simulink model "ackerman_ROS_neural_controller_v2"  (R2023a)
settings: Solver=FixedStepDiscrete  StartTime=0.0  StopTime=200  FixedStep=0.1  RelTol=1e-3
undefined symbols (not defined in the file or in its folder): Angular, Linear
libraries: neural x413, robotlib x15, robotcorelib x1
(part 15 of 17)

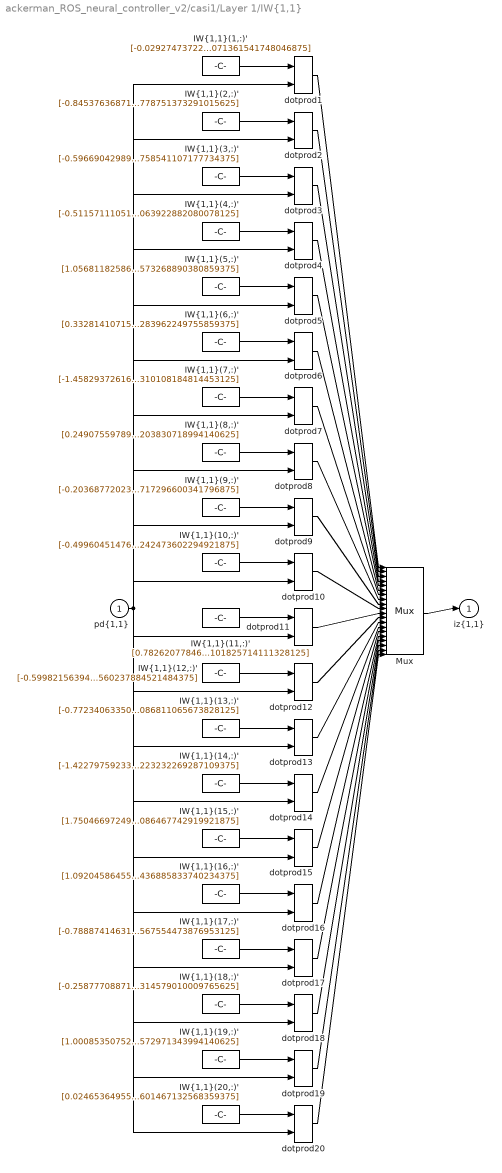
== system ackerman_ROS_neural_controller_v2/casi1/Layer 1/IW{1,1} ==
  "pd{1,1}" : Inport  PortDimensions=8  SampleTime=0.1
      mask Display: e = 0.06;c1 = [120 230 180]/255;c2 = ([120 230 180]+0)/(256+128);c3 = ([120 230 180]+128)/(256+128);patch([0 1 1 0],[0 0 1 1],c1);patch([0 1 1 1-e 1-e 0+e],[0 0 1 1-e 0+e 0+e],c2);patch([0 0 1 1-e 0+e 0+e],[0 1 1 1-e 1-e 0+e],c3);plot([0 1 1 0 0],[0 0 1 1 0]);
  "IW{1,1}(1,:)'" : Constant  Value=[-0.029274737222208684073176954143491457216441631317138671875;-1.0490069849334577867239204351790249347686767578125;-1.018709890416383156974688972695730626583099365234375;0.51758057561495485199287713840021751821041107177734375;-0.49421140001316643530770988945732824504375457763671875;-1.148479697189265014145576060400344431400299072265625;-0.1589169134791238169324145701466477476060390472412109375;-0.12069391049774129409666301171455415897071361541748046875]
      mask Display: e = 0.06;c1 = [120 150 230]/255;c2 = ([120 150 230]+0)/383;c3 = ([120 150 230]+128)/383;patch([0 1 1 0],[0 0 1 1],c1);patch([0 1 1 1-e 1-e 0+e],[0 0 1 1-e 0+e 0+e],c2);patch([0 0 1 1-e 0+e 0+e],[0 1 1 1-e 1-e 0+e],c3);plot([0 1 1 0 0],[0 0 1 1 0]);disp('Weights');
  "IW{1,1}(10,:)'" : Constant  Value=[-0.49960451476214462473990352009423077106475830078125;0.84481568535207518522156533435918390750885009765625;0.328484535401980470847860260619199834764003753662109375;1.38195060372174882701301612542010843753814697265625;-1.020587480316577977390579690109007060527801513671875;-1.05782819768129865423134106094948947429656982421875;-1.038884014221790774712417260161601006984710693359375;-0.5820201999400473891199681020225398242473602294921875]
      mask Display: e = 0.06;c1 = [120 150 230]/255;c2 = ([120 150 230]+0)/383;c3 = ([120 150 230]+128)/383;patch([0 1 1 0],[0 0 1 1],c1);patch([0 1 1 1-e 1-e 0+e],[0 0 1 1-e 0+e 0+e],c2);patch([0 0 1 1-e 0+e 0+e],[0 1 1 1-e 1-e 0+e],c3);plot([0 1 1 0 0],[0 0 1 1 0]);disp('Weights');
  "IW{1,1}(11,:)'" : Constant  Value=[0.78262077846378497181234479285194538533687591552734375;1.506770310513398936080875500920228660106658935546875;0.86605393694049992436845286647439934313297271728515625;0.0785178721101223719980310988830751739442348480224609375;-0.2140063053068555765090508202774799428880214691162109375;-2.454262585311906885721100479713641107082366943359375;1.6946832898832386860021870234049856662750244140625;-0.38077853428415864289746650683810003101825714111328125]
      mask Display: e = 0.06;c1 = [120 150 230]/255;c2 = ([120 150 230]+0)/383;c3 = ([120 150 230]+128)/383;patch([0 1 1 0],[0 0 1 1],c1);patch([0 1 1 1-e 1-e 0+e],[0 0 1 1-e 0+e 0+e],c2);patch([0 0 1 1-e 0+e 0+e],[0 1 1 1-e 1-e 0+e],c3);plot([0 1 1 0 0],[0 0 1 1 0]);disp('Weights');
  "IW{1,1}(12,:)'" : Constant  Value=[-0.599821563945515112692419279483146965503692626953125;-1.2038921753291866867385806472157128155231475830078125;0.1467090791546092898300912565900944173336029052734375;-0.9339192656969517170040262499242089688777923583984375;-1.9352619442102187985454975205357186496257781982421875;0.423900644271696436238272553964634425938129425048828125;-0.2311222652018269096974023568691336549818515777587890625;-0.432161927375341592405533219789504073560237884521484375]
      mask Display: e = 0.06;c1 = [120 150 230]/255;c2 = ([120 150 230]+0)/383;c3 = ([120 150 230]+128)/383;patch([0 1 1 0],[0 0 1 1],c1);patch([0 1 1 1-e 1-e 0+e],[0 0 1 1-e 0+e 0+e],c2);patch([0 0 1 1-e 0+e 0+e],[0 1 1 1-e 1-e 0+e],c3);plot([0 1 1 0 0],[0 0 1 1 0]);disp('Weights');
  "IW{1,1}(13,:)'" : Constant  Value=[-0.77234063350789605717494623604579828679561614990234375;-0.678866375462015891883993390365503728389739990234375;0.520805280323371366790752290398813784122467041015625;0.59851454718035934643438622515532188117504119873046875;-0.138405727580928117337322191815474070608615875244140625;-1.41761697214059267935226671397686004638671875;0.7043140607950550968752168046194128692150115966796875;-0.2470794229904558492183497264704783447086811065673828125]
      mask Display: e = 0.06;c1 = [120 150 230]/255;c2 = ([120 150 230]+0)/383;c3 = ([120 150 230]+128)/383;patch([0 1 1 0],[0 0 1 1],c1);patch([0 1 1 1-e 1-e 0+e],[0 0 1 1-e 0+e 0+e],c2);patch([0 0 1 1-e 0+e 0+e],[0 1 1 1-e 1-e 0+e],c3);plot([0 1 1 0 0],[0 0 1 1 0]);disp('Weights');
  "IW{1,1}(14,:)'" : Constant  Value=[-1.4227975923300253402459247809019871056079864501953125;0.2249135113468267721525961633233237080276012420654296875;-0.11069963821488136568316207331008627079427242279052734375;-0.287756824738865824020450645548407919704914093017578125;-0.2221314694261346256443090396714978851377964019775390625;0.87249899572179823170614554328494705259799957275390625;1.55828917261681088035629727528430521488189697265625;-0.27320712988680317945267006507492624223232269287109375]
      mask Display: e = 0.06;c1 = [120 150 230]/255;c2 = ([120 150 230]+0)/383;c3 = ([120 150 230]+128)/383;patch([0 1 1 0],[0 0 1 1],c1);patch([0 1 1 1-e 1-e 0+e],[0 0 1 1-e 0+e 0+e],c2);patch([0 0 1 1-e 0+e 0+e],[0 1 1 1-e 1-e 0+e],c3);plot([0 1 1 0 0],[0 0 1 1 0]);disp('Weights');
  "IW{1,1}(15,:)'" : Constant  Value=[1.75046697249188554224019753746688365936279296875;0.08984116482228952926814002921673818491399288177490234375;-0.95713466964004378922936666640453040599822998046875;0.7317353014971319513648495558300055563449859619140625;-2.68016820239087838473324154620058834552764892578125;-0.90201904061919024879756534573971293866634368896484375;-0.7221269694326897248259911066270433366298675537109375;0.4329605420672191229414238478057086467742919921875]
      mask Display: e = 0.06;c1 = [120 150 230]/255;c2 = ([120 150 230]+0)/383;c3 = ([120 150 230]+128)/383;patch([0 1 1 0],[0 0 1 1],c1);patch([0 1 1 1-e 1-e 0+e],[0 0 1 1-e 0+e 0+e],c2);patch([0 0 1 1-e 0+e 0+e],[0 1 1 1-e 1-e 0+e],c3);plot([0 1 1 0 0],[0 0 1 1 0]);disp('Weights');
  "IW{1,1}(16,:)'" : Constant  Value=[1.0920458645567041600088487030006945133209228515625;-0.5248332683159759870505922663141973316669464111328125;0.133055242325883560372545844074920751154422760009765625;-1.6158465686473670874789831941598094999790191650390625;0.1301728842012035425312888037296943366527557373046875;1.0353583719112287031549612947856076061725616455078125;-0.15634453093225264552756925695575773715972900390625;0.316614497875865319453936308491392992436885833740234375]
      mask Display: e = 0.06;c1 = [120 150 230]/255;c2 = ([120 150 230]+0)/383;c3 = ([120 150 230]+128)/383;patch([0 1 1 0],[0 0 1 1],c1);patch([0 1 1 1-e 1-e 0+e],[0 0 1 1-e 0+e 0+e],c2);patch([0 0 1 1-e 0+e 0+e],[0 1 1 1-e 1-e 0+e],c3);plot([0 1 1 0 0],[0 0 1 1 0]);disp('Weights');
  "IW{1,1}(17,:)'" : Constant  Value=[-0.7888741463106045959108314491459168493747711181640625;1.1072615342611840105746523477137088775634765625;0.8796331372925731972856056017917580902576446533203125;0.7814384704627406197374739349470473825931549072265625;0.50028462781930149727571688345051370561122894287109375;0.53862571872060305278040459597832523286342620849609375;0.751452913105652431369207988609559834003448486328125;-0.29818398484482433463682582441833801567554473876953125]
      mask Display: e = 0.06;c1 = [120 150 230]/255;c2 = ([120 150 230]+0)/383;c3 = ([120 150 230]+128)/383;patch([0 1 1 0],[0 0 1 1],c1);patch([0 1 1 1-e 1-e 0+e],[0 0 1 1-e 0+e 0+e],c2);patch([0 0 1 1-e 0+e 0+e],[0 1 1 1-e 1-e 0+e],c3);plot([0 1 1 0 0],[0 0 1 1 0]);disp('Weights');
  "IW{1,1}(18,:)'" : Constant  Value=[-0.258777088718072312278906110805110074579715728759765625;-1.2322924356079312246947665698826313018798828125;1.192942190263779789205500492244027554988861083984375;-1.151594999717930445370939196436665952205657958984375;-1.1499392434027362330795085654244758188724517822265625;0.259227884795615370894239504195866174995899200439453125;1.360290219702025904524589350330643355846405029296875;0.56917806478145271942281624433235265314579010009765625]
      mask Display: e = 0.06;c1 = [120 150 230]/255;c2 = ([120 150 230]+0)/383;c3 = ([120 150 230]+128)/383;patch([0 1 1 0],[0 0 1 1],c1);patch([0 1 1 1-e 1-e 0+e],[0 0 1 1-e 0+e 0+e],c2);patch([0 0 1 1-e 0+e 0+e],[0 1 1 1-e 1-e 0+e],c3);plot([0 1 1 0 0],[0 0 1 1 0]);disp('Weights');
  "IW{1,1}(19,:)'" : Constant  Value=[1.0008535075295441618692393603851087391376495361328125;-0.35035988276601326418813187046907842159271240234375;-1.02299740574121944547414386761374771595001220703125;0.415121070719786933178596655125147663056850433349609375;-1.6229572869315156413705381055478937923908233642578125;-0.1767218704602812329174099659212515689432621002197265625;-1.747820353299990525641760541475377976894378662109375;-0.036697162768480284800176605131127871572971343994140625]
      mask Display: e = 0.06;c1 = [120 150 230]/255;c2 = ([120 150 230]+0)/383;c3 = ([120 150 230]+128)/383;patch([0 1 1 0],[0 0 1 1],c1);patch([0 1 1 1-e 1-e 0+e],[0 0 1 1-e 0+e 0+e],c2);patch([0 0 1 1-e 0+e 0+e],[0 1 1 1-e 1-e 0+e],c3);plot([0 1 1 0 0],[0 0 1 1 0]);disp('Weights');
  "IW{1,1}(2,:)'" : Constant  Value=[-0.84537636871794685777814493121695704758167266845703125;-0.5251436375029034930861371321952901780605316162109375;-0.198283689819528541331550286486162804067134857177734375;-0.931487677632240274050445805187337100505828857421875;0.87292018786466629709508424639352597296237945556640625;0.3435392775267456233478924332302995026111602783203125;0.4523372398676921424254260273301042616367340087890625;1.02324209293281942478870405466295778751373291015625]
      mask Display: e = 0.06;c1 = [120 150 230]/255;c2 = ([120 150 230]+0)/383;c3 = ([120 150 230]+128)/383;patch([0 1 1 0],[0 0 1 1],c1);patch([0 1 1 1-e 1-e 0+e],[0 0 1 1-e 0+e 0+e],c2);patch([0 0 1 1-e 0+e 0+e],[0 1 1 1-e 1-e 0+e],c3);plot([0 1 1 0 0],[0 0 1 1 0]);disp('Weights');
  "IW{1,1}(20,:)'" : Constant  Value=[0.0246536495565588854861349688007976510562002658843994140625;0.722418894635240338431003692676313221454620361328125;0.308225606568565790865932285669259727001190185546875;-0.74711808212722530253557806645403616130352020263671875;0.6473758621751877218031268057529814541339874267578125;1.0113325472597025633803013988654129207134246826171875;1.2804011531948251700896435067988932132720947265625;0.81310816689997122974631338365725241601467132568359375]
      mask Display: e = 0.06;c1 = [120 150 230]/255;c2 = ([120 150 230]+0)/383;c3 = ([120 150 230]+128)/383;patch([0 1 1 0],[0 0 1 1],c1);patch([0 1 1 1-e 1-e 0+e],[0 0 1 1-e 0+e 0+e],c2);patch([0 0 1 1-e 0+e 0+e],[0 1 1 1-e 1-e 0+e],c3);plot([0 1 1 0 0],[0 0 1 1 0]);disp('Weights');
  "IW{1,1}(3,:)'" : Constant  Value=[-0.59669042989209486460566722598741762340068817138671875;-0.723519288606352173331970334402285516262054443359375;-1.19506832655980854696053938823752105236053466796875;-0.383576814027077273028254467135411687195301055908203125;0.437797254705376726047205693248542957007884979248046875;-0.2125326125783702779781236813505529426038265228271484375;0.32703293898539176343120971068856306374073028564453125;1.205944129817137167037799372337758541107177734375]
      mask Display: e = 0.06;c1 = [120 150 230]/255;c2 = ([120 150 230]+0)/383;c3 = ([120 150 230]+128)/383;patch([0 1 1 0],[0 0 1 1],c1);patch([0 1 1 1-e 1-e 0+e],[0 0 1 1-e 0+e 0+e],c2);patch([0 0 1 1-e 0+e 0+e],[0 1 1 1-e 1-e 0+e],c3);plot([0 1 1 0 0],[0 0 1 1 0]);disp('Weights');
  "IW{1,1}(4,:)'" : Constant  Value=[-0.5115711105157461080494840643950738012790679931640625;1.0521838041364703908442379542975686490535736083984375;0.50863571518541028648741075812722556293010711669921875;-1.1838398478723366480380718712694942951202392578125;-1.08411270165468831550015238462947309017181396484375;0.8662226054333241886951100241276435554027557373046875;0.84809475502056919093973874623770825564861297607421875;0.42596408239022753861036107991822063922882080078125]
      mask Display: e = 0.06;c1 = [120 150 230]/255;c2 = ([120 150 230]+0)/383;c3 = ([120 150 230]+128)/383;patch([0 1 1 0],[0 0 1 1],c1);patch([0 1 1 1-e 1-e 0+e],[0 0 1 1-e 0+e 0+e],c2);patch([0 0 1 1-e 0+e 0+e],[0 1 1 1-e 1-e 0+e],c3);plot([0 1 1 0 0],[0 0 1 1 0]);disp('Weights');
  "IW{1,1}(5,:)'" : Constant  Value=[1.0568118258682221988209448682027868926525115966796875;0.210499125407347331684349001079681329429149627685546875;1.0699205593447860263012216819333843886852264404296875;-0.1922336474073897683023659510581637732684612274169921875;-0.08614160940607092087351048803611774928867816925048828125;-0.8616777536035387097257398636429570615291595458984375;1.125359811295023160226946856710128486156463623046875;-0.439011226894258255182279526707134209573268890380859375]
      mask Display: e = 0.06;c1 = [120 150 230]/255;c2 = ([120 150 230]+0)/383;c3 = ([120 150 230]+128)/383;patch([0 1 1 0],[0 0 1 1],c1);patch([0 1 1 1-e 1-e 0+e],[0 0 1 1-e 0+e 0+e],c2);patch([0 0 1 1-e 0+e 0+e],[0 1 1 1-e 1-e 0+e],c3);plot([0 1 1 0 0],[0 0 1 1 0]);disp('Weights');
  "IW{1,1}(6,:)'" : Constant  Value=[0.332814107151104321413725983802578411996364593505859375;-1.084064403964139611247219363576732575893402099609375;-0.00061555051474618087403722910266878898255527019500732421875;1.1103898448733697801316111508640460669994354248046875;0.862902030318888346727135285618714988231658935546875;-1.053555340404520368480234537855722010135650634765625;-0.52288713379513762635752982532721944153308868408203125;-1.3744865802685450884013107497594319283962249755859375]
      mask Display: e = 0.06;c1 = [120 150 230]/255;c2 = ([120 150 230]+0)/383;c3 = ([120 150 230]+128)/383;patch([0 1 1 0],[0 0 1 1],c1);patch([0 1 1 1-e 1-e 0+e],[0 0 1 1-e 0+e 0+e],c2);patch([0 0 1 1-e 0+e 0+e],[0 1 1 1-e 1-e 0+e],c3);plot([0 1 1 0 0],[0 0 1 1 0]);disp('Weights');
  "IW{1,1}(7,:)'" : Constant  Value=[-1.4582937261694481900775599569897167384624481201171875;0.78662293007852046589079009208944626152515411376953125;-1.0577706750454367590208448746125213801860809326171875;-0.474330169066695506163711115732439793646335601806640625;1.21926975987516517108133484725840389728546142578125;-0.0305549403662195469266738001579142292030155658721923828125;-0.76767248632960105592104582683532498776912689208984375;1.1770335282473116667034673810121603310108184814453125]
      mask Display: e = 0.06;c1 = [120 150 230]/255;c2 = ([120 150 230]+0)/383;c3 = ([120 150 230]+128)/383;patch([0 1 1 0],[0 0 1 1],c1);patch([0 1 1 1-e 1-e 0+e],[0 0 1 1-e 0+e 0+e],c2);patch([0 0 1 1-e 0+e 0+e],[0 1 1 1-e 1-e 0+e],c3);plot([0 1 1 0 0],[0 0 1 1 0]);disp('Weights');
  "IW{1,1}(8,:)'" : Constant  Value=[0.2490755978917232604796794248613878153264522552490234375;-0.1421049032694032820955953866359777748584747314453125;0.418631376211793193586885308832279406487941741943359375;0.7926807121994132732112348094233311712741851806640625;1.5912523807604290748685116341221146285533905029296875;2.10200872163414853588392361416481435298919677734375;-0.285937781480293418123750370796187780797481536865234375;2.56025575206086219992585029103793203830718994140625]
      mask Display: e = 0.06;c1 = [120 150 230]/255;c2 = ([120 150 230]+0)/383;c3 = ([120 150 230]+128)/383;patch([0 1 1 0],[0 0 1 1],c1);patch([0 1 1 1-e 1-e 0+e],[0 0 1 1-e 0+e 0+e],c2);patch([0 0 1 1-e 0+e 0+e],[0 1 1 1-e 1-e 0+e],c3);plot([0 1 1 0 0],[0 0 1 1 0]);disp('Weights');
  "IW{1,1}(9,:)'" : Constant  Value=[-0.203687720234735525348668261358398012816905975341796875;-1.1673223114305810721447187461308203637599945068359375;1.5636617573684181703441709032631479203701019287109375;1.3837913949641087452135934654506854712963104248046875;-0.065402042531500781397113541970611549913883209228515625;-0.7995691008696501622665664399391971528530120849609375;-1.2460621400505071942887980185332708060741424560546875;0.044229790280105756028472541174778598360717296600341796875]
      mask Display: e = 0.06;c1 = [120 150 230]/255;c2 = ([120 150 230]+0)/383;c3 = ([120 150 230]+128)/383;patch([0 1 1 0],[0 0 1 1],c1);patch([0 1 1 1-e 1-e 0+e],[0 0 1 1-e 0+e 0+e],c2);patch([0 0 1 1-e 0+e 0+e],[0 1 1 1-e 1-e 0+e],c3);plot([0 1 1 0 0],[0 0 1 1 0]);disp('Weights');
  Mux : Mux  Inputs=20
      mask Display: e = 0.06;c1 = [120 150 230]/255;c2 = ([120 150 230]+0)/383;c3 = ([120 150 230]+128)/383;patch([0 1 1 0],[0 0 1 1],c1);patch([0 1 1 1-e 1-e 0+e],[0 0 1 1-e 0+e 0+e],c2);patch([0 0 1 1-e 0+e 0+e],[0 1 1 1-e 1-e 0+e],c3);plot([0 1 1 0 0],[0 0 1 1 0]);disp('Mux');
  dotprod{1..20} (20 alike) : neural/Weight Functions/dotprod
  "iz{1,1}" : Outport
      mask Display: e = 0.06;c1 = [120 230 180]/255;c2 = ([120 230 180]+0)/(256+128);c3 = ([120 230 180]+128)/(256+128);patch([0 1 1 0],[0 0 1 1],c1);patch([0 1 1 1-e 1-e 0+e],[0 0 1 1-e 0+e 0+e],c2);patch([0 0 1 1-e 0+e 0+e],[0 1 1 1-e 1-e 0+e],c3);plot([0 1 1 0 0],[0 0 1 1 0]);
  wires:
  "IW{1,1}(1,:)'"/1 -> dotprod1/1
  "pd{1,1}"/1 -> dotprod1/2, dotprod2/2, dotprod3/2, dotprod4/2, dotprod5/2, dotprod6/2, dotprod7/2, dotprod8/2, dotprod9/2, dotprod10/2, dotprod11/2, dotprod12/2, dotprod13/2, dotprod14/2, dotprod15/2, dotprod16/2, dotprod17/2, dotprod18/2, dotprod19/2, dotprod20/2
  dotprod1/1 -> Mux/1
  "IW{1,1}(2,:)'"/1 -> dotprod2/1
  dotprod2/1 -> Mux/2
  "IW{1,1}(3,:)'"/1 -> dotprod3/1
  dotprod3/1 -> Mux/3
  "IW{1,1}(4,:)'"/1 -> dotprod4/1
  dotprod4/1 -> Mux/4
  "IW{1,1}(5,:)'"/1 -> dotprod5/1
  dotprod5/1 -> Mux/5
  "IW{1,1}(6,:)'"/1 -> dotprod6/1
  dotprod6/1 -> Mux/6
  "IW{1,1}(7,:)'"/1 -> dotprod7/1
  dotprod7/1 -> Mux/7
  "IW{1,1}(8,:)'"/1 -> dotprod8/1
  dotprod8/1 -> Mux/8
  "IW{1,1}(9,:)'"/1 -> dotprod9/1
  dotprod9/1 -> Mux/9
  "IW{1,1}(10,:)'"/1 -> dotprod10/1
  dotprod10/1 -> Mux/10
  "IW{1,1}(11,:)'"/1 -> dotprod11/1
  dotprod11/1 -> Mux/11
  "IW{1,1}(12,:)'"/1 -> dotprod12/1
  dotprod12/1 -> Mux/12
  "IW{1,1}(13,:)'"/1 -> dotprod13/1
  dotprod13/1 -> Mux/13
  "IW{1,1}(14,:)'"/1 -> dotprod14/1
  dotprod14/1 -> Mux/14
  "IW{1,1}(15,:)'"/1 -> dotprod15/1
  dotprod15/1 -> Mux/15
  "IW{1,1}(16,:)'"/1 -> dotprod16/1
  dotprod16/1 -> Mux/16
  "IW{1,1}(17,:)'"/1 -> dotprod17/1
  dotprod17/1 -> Mux/17
  "IW{1,1}(18,:)'"/1 -> dotprod18/1
  dotprod18/1 -> Mux/18
  "IW{1,1}(19,:)'"/1 -> dotprod19/1
  dotprod19/1 -> Mux/19
  "IW{1,1}(20,:)'"/1 -> dotprod20/1
  dotprod20/1 -> Mux/20
  Mux/1 -> "iz{1,1}"/1

== system ackerman_ROS_neural_controller_v2/casi1/Layer 2/Delays 1 ==
  "p{2}" : Inport  PortDimensions=20  SampleTime=0.1
      mask Display: e = 0.06;c1 = [120 230 180]/255;c2 = ([120 230 180]+0)/(256+128);c3 = ([120 230 180]+128)/(256+128);patch([0 1 1 0],[0 0 1 1],c1);patch([0 1 1 1-e 1-e 0+e],[0 0 1 1-e 0+e 0+e],c2);patch([0 0 1 1-e 0+e 0+e],[0 1 1 1-e 1-e 0+e],c3);plot([0 1 1 0 0],[0 0 1 1 0]);
  mux : Mux  Inputs=1
      mask Display: e = 0.06;c1 = [120 150 230]/255;c2 = ([120 150 230]+0)/383;c3 = ([120 150 230]+128)/383;patch([0 1 1 0],[0 0 1 1],c1);patch([0 1 1 1-e 1-e 0+e],[0 0 1 1-e 0+e 0+e],c2);patch([0 0 1 1-e 0+e 0+e],[0 1 1 1-e 1-e 0+e],c3);plot([0 1 1 0 0],[0 0 1 1 0]);disp('Mux')
  "pd{2,1}" : Outport
      mask Display: e = 0.06;c1 = [120 230 180]/255;c2 = ([120 230 180]+0)/(256+128);c3 = ([120 230 180]+128)/(256+128);patch([0 1 1 0],[0 0 1 1],c1);patch([0 1 1 1-e 1-e 0+e],[0 0 1 1-e 0+e 0+e],c2);patch([0 0 1 1-e 0+e 0+e],[0 1 1 1-e 1-e 0+e],c3);plot([0 1 1 0 0],[0 0 1 1 0]);
  wires:
  "p{2}"/1 -> mux/1
  mux/1 -> "pd{2,1}"/1
